simulink model "Ytest_R2023a"  (R2023a)
settings: Solver=VariableStepAuto  StartTime=0.0  StopTime=0.1  RelTol=1e-3  AbsTol=1e-3  EnableMultiTasking=on
values from neighbouring files (symbols this model uses):
  C2 = 100e-6    (= 0.0001)    [Sim_Yest.m]
  L = 200e-6    (= 0.0002)    [Sim_Yest.m]
  Nsw = 1    [Sim_Yest.m]
  P1sw = 0    [Sim_Yest.m]
  P2sw = 0    [Sim_Yest.m]
  Ra = 50e-3    (= 0.05)    [Sim_Yest.m]
  sample_time = 1e-6    (= 1e-06)    [Sim_Yest.m]
  Vdc = 800    [Sim_Yest.m]
libraries: spsMosfetLib x15, spsCurrentMeasurementLib x5, spsSeriesRLCBranchLib x4, spsTriangleGeneratorLib x2, spsVoltageMeasurementLib x2, spsDCVoltageSourceLib x1, spsGroundLib x1, spspowerguiLib x1
settings Model: Creator=snow_  LastModifiedBy=snow_
settings SolverCC: AutoScaleAbsTol=off  AlgebraicLoopSolver=TrustRegion
settings DataIOCC: LimitDataPoints=on  MaxDataPoints=10000  ReturnWorkspaceOutputs=off
settings OptimizationCC: LifeSpan=inf
settings DebuggingCC: UnconnectedInputMsg=warning  UnconnectedOutputMsg=warning  UnconnectedLineMsg=warning  AllowSymbolicDim=off  SFUnexpectedBacktrackingDiag=warning  SFNoUnconditionalDefaultTransitionDiag=warning  SFExecutionAtInitializationDiag=none  ArithmeticOperatorsInVariantConditions=warning
settings ModelReferenceCC: EnableRefExpFcnMdlSchedulingChecks=on
settings SFSimCC: SimUseLocalCustomCode=off  CustomCodeUndefinedFunction=UseInterfaceOnly
settings RTWCC: RTWUseLocalCustomCode=off
settings CodeAppCC: StateflowObjectComments=on
settings GRTTargetCC: TargetLangStandard=C89/C90 (ANSI)
settings ConfigComp: CovMetricSettings=dw  CovSaveCumulativeToWorkspaceVar=on  CovSaveSingleToWorkspaceVar=on  CovExternalEMLEnable=off  CovSFcnEnable=off
settings SimscapeCC: SimscapeLogType=all  SimscapeLogDataHistory=10000

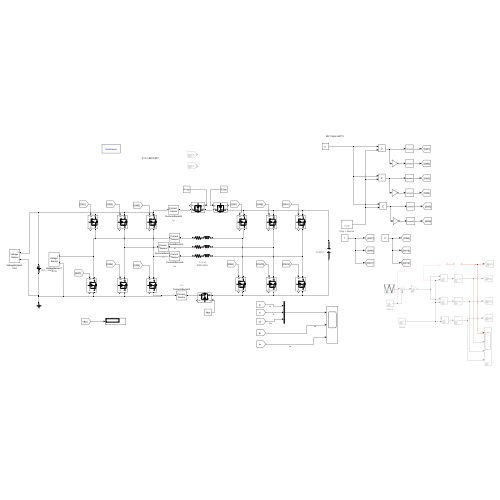
[thumbnail: Simulink's stored preview of the top-level diagram]
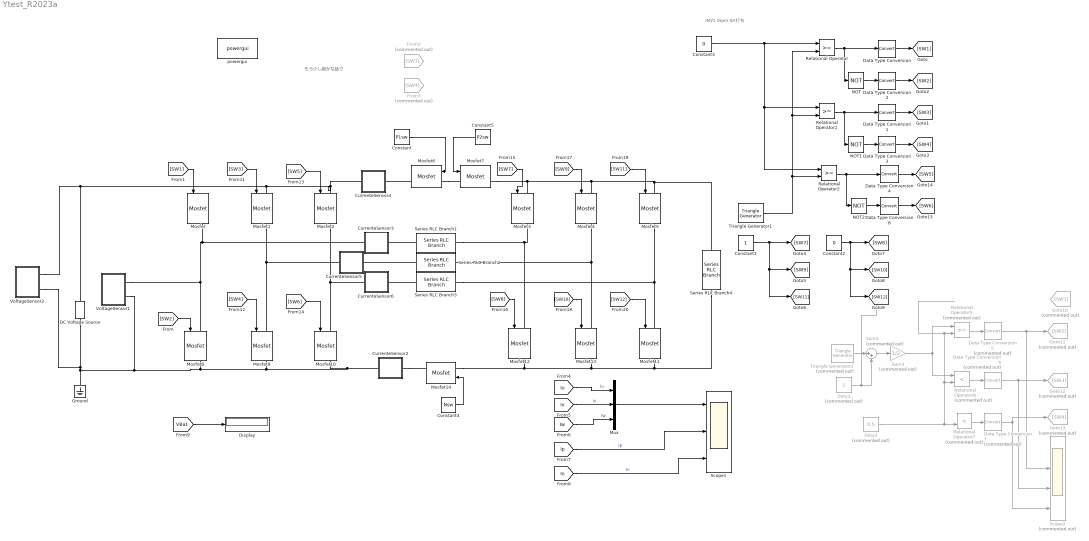
== system Ytest_R2023a ==
  note: INV1 0rpm 0A打ち
  note: もう少し細かな話で
  Constant : Constant  Value=P1sw
  Constant1 : Constant
  Constant2 : Constant  Value=0
  Constant3 : Constant  Value=0
  Constant4 : Constant  Value=Nsw
  Constant5 : Constant  Value=P2sw
  CurrenteSensor2 : Subsystem  mask{VariableName=In, SampleTime=sample_time}
      mask prompts: VariableName "Simulink:blkprm_prompts:ToWksVarName"
      settings: AttributesFormatString=%<VariableName>
      mask TypeOptions VariableName: To Workspace1/VariableName | Goto/GotoTag
      mask DialogControl VariableName Prompt: 変数名:
      mask Display:
      | disp("Current \n Sensor")
      | port_label('lconn', 1, '+')
      | port_label('rconn', 1, '-')
      | 
      | 
      | %set_param([gcb '/Goto'],'GotoTag',VariableName) % これは使えないっぽい
  CurrenteSensor3 : Subsystem  mask{VariableName=Iu, SampleTime=sample_time}
      mask prompts: VariableName "Simulink:blkprm_prompts:ToWksVarName"
      settings: AttributesFormatString=%<VariableName>
      mask TypeOptions VariableName: To Workspace1/VariableName | Goto/GotoTag
      mask DialogControl VariableName Prompt: 変数名:
      mask Display:
      | disp("Current \n Sensor")
      | port_label('lconn', 1, '+')
      | port_label('rconn', 1, '-')
      | 
      | 
      | %set_param([gcb '/Goto'],'GotoTag',VariableName) % これは使えないっぽい
  CurrenteSensor4 : Subsystem  mask{VariableName=Ip, SampleTime=sample_time}
      mask prompts: VariableName "Simulink:blkprm_prompts:ToWksVarName"
      settings: AttributesFormatString=%<VariableName>
      mask TypeOptions VariableName: To Workspace1/VariableName | Goto/GotoTag
      mask DialogControl VariableName Prompt: 変数名:
      mask Display:
      | disp("Current \n Sensor")
      | port_label('lconn', 1, '+')
      | port_label('rconn', 1, '-')
      | 
      | 
      | %set_param([gcb '/Goto'],'GotoTag',VariableName) % これは使えないっぽい
  CurrenteSensor5 : Subsystem  mask{VariableName=Iv, SampleTime=sample_time}
      mask prompts: VariableName "Simulink:blkprm_prompts:ToWksVarName"
      settings: AttributesFormatString=%<VariableName>
      mask TypeOptions VariableName: To Workspace1/VariableName | Goto/GotoTag
      mask DialogControl VariableName Prompt: 変数名:
      mask Display:
      | disp("Current \n Sensor")
      | port_label('lconn', 1, '+')
      | port_label('rconn', 1, '-')
      | 
      | 
      | %set_param([gcb '/Goto'],'GotoTag',VariableName) % これは使えないっぽい
  CurrenteSensor6 : Subsystem  mask{VariableName=Iw, SampleTime=sample_time}
      mask prompts: VariableName "Simulink:blkprm_prompts:ToWksVarName"
      settings: AttributesFormatString=%<VariableName>
      mask TypeOptions VariableName: To Workspace1/VariableName | Goto/GotoTag
      mask DialogControl VariableName Prompt: 変数名:
      mask Display:
      | disp("Current \n Sensor")
      | port_label('lconn', 1, '+')
      | port_label('rconn', 1, '-')
      | 
      | 
      | %set_param([gcb '/Goto'],'GotoTag',VariableName) % これは使えないっぽい
  DC Voltage Source : spsDCVoltageSourceLib/DC Voltage Source  Amplitude=Vdc  Measurements=None
      settings: AttributesFormatString=DC = %<Amplitude> V
  Data Type Conversion{,1..4,8} (6 alike) : DataTypeConversion  SaturateOnIntegerOverflow=off  RndMeth=Floor
  Data Type Conversion5 : DataTypeConversion  Commented=on  SaturateOnIntegerOverflow=off  RndMeth=Floor
  Data Type Conversion6 : DataTypeConversion  Commented=on  SaturateOnIntegerOverflow=off  RndMeth=Floor
  Data Type Conversion7 : DataTypeConversion  Commented=on  SaturateOnIntegerOverflow=off  RndMeth=Floor
  Display : Display
  Duty2 : Constant  Commented=on  Value=0.5
  Duty3 : Constant  Commented=on
  From2 : From  Commented=on  GotoTag=SW3
  From3 : From  Commented=on  GotoTag=SW4
  Gain3 : Gain  Commented=on  Gain=1/2
  Goto10 : Goto  Commented=on  GotoTag=SW1
  Goto11 : Goto  Commented=on  GotoTag=SW2
  Goto12 : Goto  Commented=on  GotoTag=SW3
  Goto13 : Goto  Commented=on  GotoTag=SW4
  Ground : spsGroundLib/Ground  LConnTagsString=a
  Mosfet{,1..14} (15 alike) : spsMosfetLib/Mosfet  Ron=0.1  Lon=0  Rd=0.01  Vfd=0  IC=0  Rs=1e5  Cs=inf  Measurements=on
  Mux : Mux  Inputs=3
  NOT : Logic  Operator=NOT  IconShape=distinctive  AllPortsSameDT=off  OutDataTypeStr=boolean
  NOT1 : Logic  Operator=NOT  IconShape=distinctive  AllPortsSameDT=off  OutDataTypeStr=boolean
  NOT2 : Logic  Operator=NOT  IconShape=distinctive  AllPortsSameDT=off  OutDataTypeStr=boolean
  Relational Operator : RelationalOperator  OutDataTypeStr=boolean  RndMeth=Simplest  InputSameDT=off
  Relational Operator1 : RelationalOperator  OutDataTypeStr=boolean  RndMeth=Simplest  InputSameDT=off
  Relational Operator2 : RelationalOperator  OutDataTypeStr=boolean  RndMeth=Simplest  InputSameDT=off
  Relational Operator5 : RelationalOperator  Commented=on  OutDataTypeStr=boolean  RndMeth=Simplest  InputSameDT=off
  Relational Operator6 : RelationalOperator  Commented=on  Operator=<  OutDataTypeStr=boolean  RndMeth=Simplest  InputSameDT=off
  Relational Operator7 : RelationalOperator  Commented=on  Operator=<  OutDataTypeStr=boolean  RndMeth=Simplest  InputSameDT=off
  Scope1 : Scope  NumInputPorts=3
  Scope2 : Scope  Commented=on  NumInputPorts=4
  Series RLC Branch1 : spsSeriesRLCBranchLib/Series RLC Branch  LConnTagsString=__new0  RConnTagsString=__new0  BranchType=RL  Resistance=Ra  Inductance=L  SetiL0=off  InitialCurrent=0  Capacitance=1e-6  Setx0=off  InitialVoltage=0  Measurements=None
      settings: AttributesFormatString=|
      | L=%<Inductance> H
      | R=%<Resistance> Ohm
  Series RLC Branch2 : spsSeriesRLCBranchLib/Series RLC Branch  LConnTagsString=__new0  RConnTagsString=__new0  BranchType=RL  Resistance=Ra  Inductance=L  SetiL0=off  InitialCurrent=0  Capacitance=1e-6  Setx0=off  InitialVoltage=0  Measurements=None
      settings: AttributesFormatString=|
      | L=%<Inductance> H
      | R=%<Resistance> Ohm
  Series RLC Branch3 : spsSeriesRLCBranchLib/Series RLC Branch  LConnTagsString=__new0  RConnTagsString=__new0  BranchType=RL  Resistance=Ra  Inductance=L  SetiL0=off  InitialCurrent=0  Capacitance=1e-6  Setx0=off  InitialVoltage=0  Measurements=None
      settings: AttributesFormatString=|
      | L=%<Inductance> H
      | R=%<Resistance> Ohm
  Series RLC Branch4 : spsSeriesRLCBranchLib/Series RLC Branch  LConnTagsString=__new0  RConnTagsString=__new0  BranchType=C  Resistance=50e-3  Inductance=200e-6  SetiL0=off  InitialCurrent=0  Capacitance=C2  Setx0=off  InitialVoltage=0  Measurements=None
      settings: AttributesFormatString=C=%<Capacitance> F
  Sum3 : Sum  Commented=on  Inputs=|++
  Triangle Generator1 : spsTriangleGeneratorLib/Triangle Generator  Freq=Fsw  Phase=0  Ts=0
      settings: AttributesFormatString=Freq = %<Freq> Hz
  Triangle Generator3 : spsTriangleGeneratorLib/Triangle Generator  Commented=on  Freq=10e3  Phase=180  Ts=0
  VoltageSensor1 : Subsystem  mask{VariableName=Vu1N, SampleTime=sample_time}
      mask prompts: VariableName "Simulink:blkprm_prompts:ToWksVarName"
      settings: AttributesFormatString=%<VariableName>
      mask TypeOptions VariableName: To Workspace1/VariableName | Goto/GotoTag
      mask DialogControl VariableName Prompt: 変数名:
      mask Display:
      | disp("Voltage \n Sensor")
      | port_label('lconn', 1, '+')
      | port_label('lconn', 2, '-')
      | 
      | 
      | %set_param([gcb '/Goto'],'GotoTag',VariableName) % これは使えないっぽい
  VoltageSensor2 : Subsystem  mask{VariableName=VBat, SampleTime=sample_time}
      mask prompts: VariableName "Simulink:blkprm_prompts:ToWksVarName"
      settings: AttributesFormatString=%<VariableName>
      mask TypeOptions VariableName: To Workspace1/VariableName | Goto/GotoTag
      mask DialogControl VariableName Prompt: 変数名:
      mask Display:
      | disp("Voltage \n Sensor")
      | port_label('lconn', 1, '+')
      | port_label('lconn', 2, '-')
      | 
      | 
      | %set_param([gcb '/Goto'],'GotoTag',VariableName) % これは使えないっぽい
  powergui : spspowerguiLib/powergui  Priority=1  SimulationMode=Continuous  SampleTime=50e-6  frequency=60  Iterations=50  frequencyindice=0  Pbase=100e6  ErrMax=1e-4  UnitsV=kV  UnitsW=MW  buscounter=0  FunctionMessages=off  echomessages=off  EnableUseOfTLC=off  CurrentSourceSwitches=off  DisableSnubberDevices=off  DisableRonSwitches=off  DisableVfSwitches=off  DisplayEquations=off  AutomaticDiscreteSolvers=off  SolverType=Tustin/Backward Euler (TBE)  Interpol=off  ExternalGateDelay=off  methode=off  Ts=100  x0status=blocks  SPID=on  SwTol=0  HookPort=off  NonlinearTolerance=1e-4  nMaxIteration=100  ContinueOnMaxIteration=off  RestoreLinks=warning  ResistiveCurrentMeasurement=off  Frange=[0:2:500]  Ylog=off  Xlog=on  ShowGrid=off  save=off  variable=ZData  structure=0  ZoomFFT=off  StartTime=0.0  cycles=1  DisplayStyle=1  fundamental=60  FreqAxis=off  MaxFrequency=1000  frequencyindicesteady=1  RmsSteady=1  display=off
  wires:
  Relational Operator/1 -> NOT/1, Data Type Conversion/1
  [SW2] -> Mosfet8/1
  Data Type Conversion/1 -> [SW1]
  [SW1] -> Mosfet/1
  ? -> Scope2/1, Goto10/1
  Duty3/1 -> Sum3/2
  Triangle Generator3/1 -> Sum3/1
  Data Type Conversion7/1 -> Goto13/1, Scope2/4
  Data Type Conversion5/1 -> Scope2/2, Goto11/1
  Sum3/1 -> Gain3/1
  Duty2/1 -> Relational Operator5/2, Relational Operator6/2, Relational Operator7/2
  Relational Operator7/1 -> Data Type Conversion7/1
  Relational Operator5/1 -> Data Type Conversion5/1
  ? -> ?
  Data Type Conversion6/1 -> Scope2/3, Goto12/1
  Gain3/1 -> Relational Operator6/1, Relational Operator5/1
  Relational Operator6/1 -> Data Type Conversion6/1
  Constant3/1 -> Relational Operator2/1, Relational Operator1/1, Relational Operator/1
  [SW4] -> Mosfet9/1
  [SW3] -> Mosfet1/1
  Constant/1 -> Mosfet6/1
  [SW8] -> Mosfet12/1
  [SW10] -> Mosfet13/1
  [SW12] -> Mosfet11/1
  [SW7] -> Mosfet3/1
  [SW9] -> Mosfet4/1
  [SW11] -> Mosfet5/1
  [SW6] -> Mosfet10/1
  [SW5] -> Mosfet2/1
  Constant2/1 -> [SW12], [SW10], [SW8]
  Constant1/1 -> [SW11], [SW9], [SW7]
  NOT/1 -> Data Type Conversion2/1
  Data Type Conversion2/1 -> [SW2]
  NOT1/1 -> Data Type Conversion3/1
  Data Type Conversion1/1 -> [SW3]
  Relational Operator1/1 -> NOT1/1, Data Type Conversion1/1
  Data Type Conversion3/1 -> [SW4]
  Relational Operator2/1 -> NOT2/1, Data Type Conversion4/1
  Data Type Conversion4/1 -> [SW5]
  Data Type Conversion8/1 -> [SW6]
  NOT2/1 -> Data Type Conversion8/1
  Triangle Generator1/1 -> Relational Operator/2, Relational Operator1/2, Relational Operator2/2
  [Iu] -> Mux/1  "Iu"
  [Iv] -> Mux/2  "Iv"
  [Iw] -> Mux/3  "Iw"
  Mux/1 -> Scope1/1
  [Ip] -> Scope1/2  "Ip"
  [In] -> Scope1/3  "In"
  [VBat] -> Display/1
  Constant4/1 -> Mosfet14/1
  Constant5/1 -> Mosfet7/1
  connections:
  Series RLC Branch4/RConn1 -- Mosfet14/LConn1 -- Mosfet12/RConn1 -- Mosfet13/RConn1 -- Mosfet11/RConn1
  Mosfet/RConn1 -- VoltageSensor1/LConn1 -- Mosfet8/LConn1 -- CurrenteSensor3/LConn1
  VoltageSensor2/LConn1 -- DC Voltage Source/RConn1 -- Mosfet1/LConn1 -- CurrenteSensor4/LConn1 -- Mosfet2/LConn1
  Mosfet1/RConn1 -- Mosfet9/LConn1 -- CurrenteSensor5/LConn1
  Mosfet2/RConn1 -- Mosfet10/LConn1 -- CurrenteSensor6/LConn1
  Mosfet4/RConn1 -- Series RLC Branch2/RConn1 -- Mosfet13/LConn1
  Mosfet5/RConn1 -- Mosfet11/LConn1 -- Series RLC Branch3/RConn1
  Mosfet6/LConn1 -- Mosfet7/LConn1
  Mosfet7/RConn1 -- Series RLC Branch4/LConn1 -- Mosfet5/LConn1 -- Mosfet4/LConn1 -- Mosfet3/LConn1
  Series RLC Branch1/RConn1 -- Mosfet12/LConn1 -- Mosfet3/RConn1
  VoltageSensor2/LConn2 -- Mosfet10/RConn1 -- CurrenteSensor2/RConn1 -- Mosfet9/RConn1 -- Mosfet8/RConn1 -- VoltageSensor1/LConn2 -- Ground/LConn1 -- DC Voltage Source/LConn1
  Mosfet6/RConn1 -- CurrenteSensor4/RConn1
  Series RLC Branch1/LConn1 -- CurrenteSensor3/RConn1
  Series RLC Branch2/LConn1 -- CurrenteSensor5/RConn1
  Series RLC Branch3/LConn1 -- CurrenteSensor6/RConn1
  CurrenteSensor2/LConn1 -- Mosfet14/RConn1

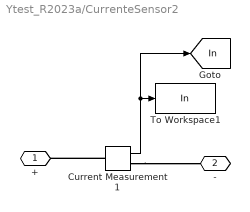
== system Ytest_R2023a/CurrenteSensor2 ==
  Current Measurement1 : spsCurrentMeasurementLib/Current Measurement  PhasorSimulation=off  OutputType=Complex  PSBequivalent=0
  To Workspace1 : ToWorkspace  VariableName=In  SampleTime=SampleTime
  + : PMIOPort  Side=Left
  - : PMIOPort  Port=2  Side=Right
  tag scope: In=global
  wires:
  Current Measurement1/1 -> [In], To Workspace1/1
  connections:
  Current Measurement1/LConn1 -- +/RConn1
  Current Measurement1/RConn1 -- -/RConn1

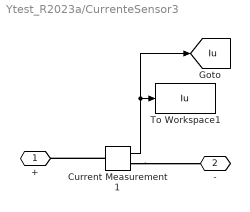
== system Ytest_R2023a/CurrenteSensor3 ==
  Current Measurement1 : spsCurrentMeasurementLib/Current Measurement  PhasorSimulation=off  OutputType=Complex  PSBequivalent=0
  To Workspace1 : ToWorkspace  VariableName=Iu  SampleTime=SampleTime
  + : PMIOPort  Side=Left
  - : PMIOPort  Port=2  Side=Right
  tag scope: Iu=global
  wires:
  Current Measurement1/1 -> [Iu], To Workspace1/1
  connections:
  Current Measurement1/LConn1 -- +/RConn1
  Current Measurement1/RConn1 -- -/RConn1

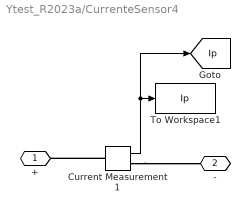
== system Ytest_R2023a/CurrenteSensor4 ==
  Current Measurement1 : spsCurrentMeasurementLib/Current Measurement  PhasorSimulation=off  OutputType=Complex  PSBequivalent=0
  To Workspace1 : ToWorkspace  VariableName=Ip  SampleTime=SampleTime
  + : PMIOPort  Side=Left
  - : PMIOPort  Port=2  Side=Right
  tag scope: Ip=global
  wires:
  Current Measurement1/1 -> [Ip], To Workspace1/1
  connections:
  Current Measurement1/LConn1 -- +/RConn1
  Current Measurement1/RConn1 -- -/RConn1

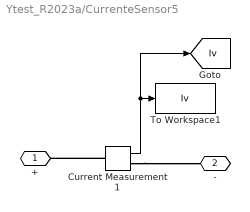
== system Ytest_R2023a/CurrenteSensor5 ==
  Current Measurement1 : spsCurrentMeasurementLib/Current Measurement  PhasorSimulation=off  OutputType=Complex  PSBequivalent=0
  To Workspace1 : ToWorkspace  VariableName=Iv  SampleTime=SampleTime
  + : PMIOPort  Side=Left
  - : PMIOPort  Port=2  Side=Right
  tag scope: Iv=global
  wires:
  Current Measurement1/1 -> [Iv], To Workspace1/1
  connections:
  Current Measurement1/LConn1 -- +/RConn1
  Current Measurement1/RConn1 -- -/RConn1

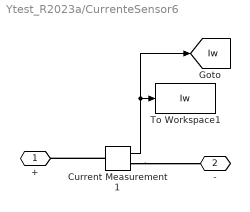
== system Ytest_R2023a/CurrenteSensor6 ==
  Current Measurement1 : spsCurrentMeasurementLib/Current Measurement  PhasorSimulation=off  OutputType=Complex  PSBequivalent=0
  To Workspace1 : ToWorkspace  VariableName=Iw  SampleTime=SampleTime
  + : PMIOPort  Side=Left
  - : PMIOPort  Port=2  Side=Right
  tag scope: Iw=global
  wires:
  Current Measurement1/1 -> [Iw], To Workspace1/1
  connections:
  Current Measurement1/LConn1 -- +/RConn1
  Current Measurement1/RConn1 -- -/RConn1

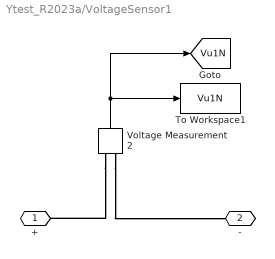
== system Ytest_R2023a/VoltageSensor1 ==
  To Workspace1 : ToWorkspace  VariableName=Vu1N  SampleTime=SampleTime
  Voltage Measurement2 : spsVoltageMeasurementLib/Voltage Measurement  PhasorSimulation=off  OutputType=Complex  PSBequivalent=0
  + : PMIOPort  Side=Left
  - : PMIOPort  Port=2  Side=Left
  tag scope: Vu1N=global
  wires:
  Voltage Measurement2/1 -> [Vu1N], To Workspace1/1
  connections:
  Voltage Measurement2/LConn1 -- +/RConn1
  Voltage Measurement2/LConn2 -- -/RConn1

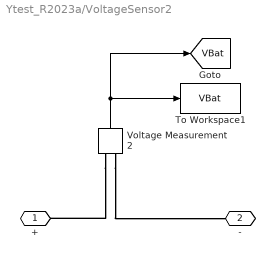
== system Ytest_R2023a/VoltageSensor2 ==
  To Workspace1 : ToWorkspace  VariableName=VBat  SampleTime=SampleTime
  Voltage Measurement2 : spsVoltageMeasurementLib/Voltage Measurement  PhasorSimulation=off  OutputType=Complex  PSBequivalent=0
  + : PMIOPort  Side=Left
  - : PMIOPort  Port=2  Side=Left
  tag scope: VBat=global
  wires:
  Voltage Measurement2/1 -> [VBat], To Workspace1/1
  connections:
  Voltage Measurement2/LConn1 -- +/RConn1
  Voltage Measurement2/LConn2 -- -/RConn1
